simulink model "Prob1_2_simulink"  (Simulink 9.3)
settings: Solver=ode45  StartTime=0.0  StopTime=tfinal  RelTol=1e-6  EnableMultiTasking=on
values from neighbouring files (symbols this model uses):
  Ap = 1.2    [Prob1_2.m]    (also in main.m)
  Bp = 1    [Prob1_2.m]    (also in main.m)
  Cp = 1    [Prob1_2.m]    (also in main.m)
  Dp = 0    [Prob1_2.m]    (also in main.m)
  h = 0.1    [Prob1_2.m]    (also in main.m)
  md = MPCInit(Ad,Bd,Cyd,Czd,Dzd,Ccd,Dcd,Hp,Hw,zblk,Hu,ublk,  	    du_max,du_min,u_max,u_min,z_max,  	    z_min,Q,R,W,V,h,cmode,solver)    [Prob1_2.m]    (also in main.m = MPCInit(Ad,Bd,Cyd,Czd,Dzd,Ccd,Dcd,Hp,Hw,zblk,Hu,ublk,       )
settings Model: Creator=jakesson  LastModifiedBy=tomas  ExtModeAutoUpdateStatusClock=off
settings DataIOCC: LimitDataPoints=on  SignalLoggingName=sigsOut
settings OptimizationCC: BooleanDataType=off  InitFltsAndDblsToZero=on
settings DebuggingCC: SaveWithParameterizedLinksMsg=none  SignalResolutionControl=TryResolveAllWithWarning  MultiTaskDSMMsg=warning  MultiTaskCondExecSysMsg=none
settings HardwareCC: TargetUnknown=on
settings GRTTargetCC: TargetFcnLib=ansi_tfl_tmw.mat  GeneratePreprocessorConditionals=Disable all

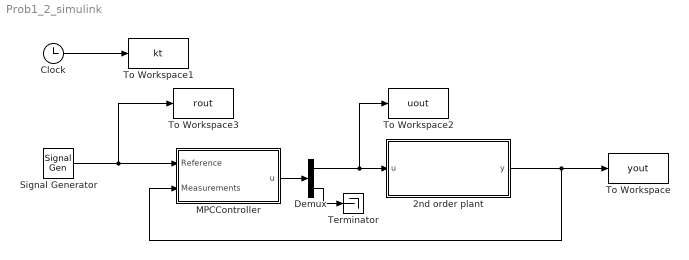
== system Prob1_2_simulink ==
  2nd order plant : Subsystem
  Clock : Clock
  Demux : Demux  Outputs=[md.m md.ne]
  MPCController : Subsystem  mask{md=md}
      mask prompts: md "MPCData"
  Signal Generator : SignalGenerator  WaveForm=square  Units=rad/sec
  Terminator : Terminator
  To Workspace : ToWorkspace  VariableName=yout  SampleTime=-1
  To Workspace1 : ToWorkspace  VariableName=kt  SampleTime=-1
  To Workspace2 : ToWorkspace  VariableName=uout  SampleTime=-1
  To Workspace3 : ToWorkspace  VariableName=rout  SampleTime=-1
  wires:
  2nd order plant/1(y) -> MPCController/2(Measurements), To Workspace/1
  Demux/2 -> Terminator/1
  MPCController/1(u) -> Demux/1
  Clock/1 -> To Workspace1/1
  Demux/1 -> 2nd order plant/1(u), To Workspace2/1
  Signal Generator/1 -> To Workspace3/1, MPCController/1(Reference)

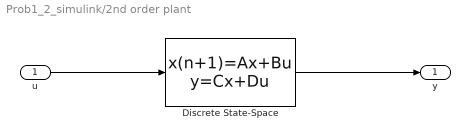
== system Prob1_2_simulink/2nd order plant ==
  u : Inport
  Discrete State-Space : DiscreteStateSpace  A=Ap  B=Bp  C=Cp  D=Dp  SampleTime=h
  y : Outport
  wires:
  Discrete State-Space/1 -> y/1
  u/1 -> Discrete State-Space/1

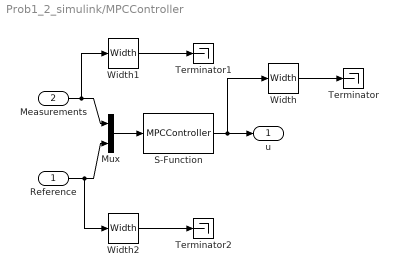
== system Prob1_2_simulink/MPCController ==
  Reference : Inport
  Measurements : Inport  Port=2
  Mux : Mux  Inputs=2
  S-Function : S-Function  FunctionName=MPCController  Parameters=md  SFunctionDeploymentMode=off  EnableBusSupport=off
  Terminator : Terminator
  Terminator1 : Terminator
  Terminator2 : Terminator
  Width : Width
  Width1 : Width
  Width2 : Width
  u : Outport
  wires:
  Mux/1 -> S-Function/1
  Measurements/1 -> Width1/1, Mux/1
  Reference/1 -> Width2/1, Mux/2
  S-Function/1 -> Width/1, u/1
  Width/1 -> Terminator/1
  Width1/1 -> Terminator1/1
  Width2/1 -> Terminator2/1
